simulink model "Blood_Pressure(Wrong)"  (R2024b)
settings: Solver=VariableStepAuto  StartTime=0.0  StopTime=10.0  RelTol=1e-3
values from neighbouring files (symbols this model uses):
  Ca = 87.5    [Blood_Pressure_Model.m]
  Co = 80    [Blood_Pressure_Model.m]
  MAP = 82.5    [Blood_Pressure_Model.m]
  VO2 = 37.5    [Blood_Pressure_Model.m]
undefined symbols (not defined in the file or in its folder): CVP
settings Model: Creator=Stephon Woodson  LastModifiedBy=Stephon Woodson

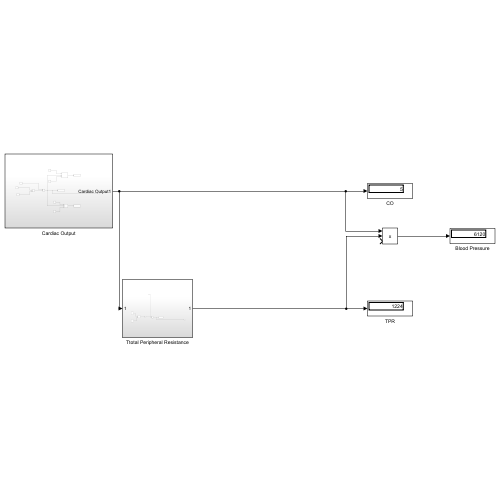
[thumbnail: Simulink's stored preview of the top-level diagram]
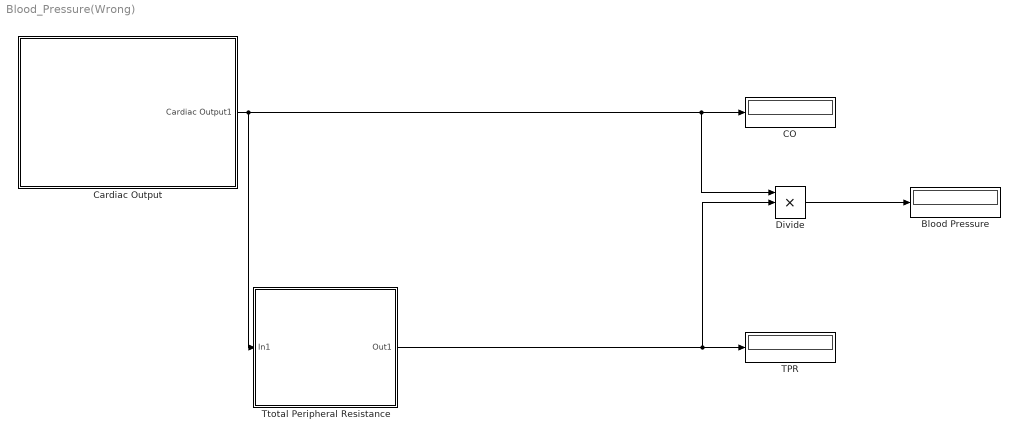
== system Blood_Pressure(Wrong) ==
  Blood Pressure : Display
  CO : Display
  Cardiac Output : Subsystem
  Divide : Product  Inputs=***
  TPR : Display
  Ttotal Peripheral Resistance : Subsystem
  wires:
  Cardiac Output/1(Cardiac Output1) -> Ttotal Peripheral Resistance/1(In1), Divide/1, CO/1
  Ttotal Peripheral Resistance/1(Out1) -> Divide/2, TPR/1
  Divide/1 -> Blood Pressure/1

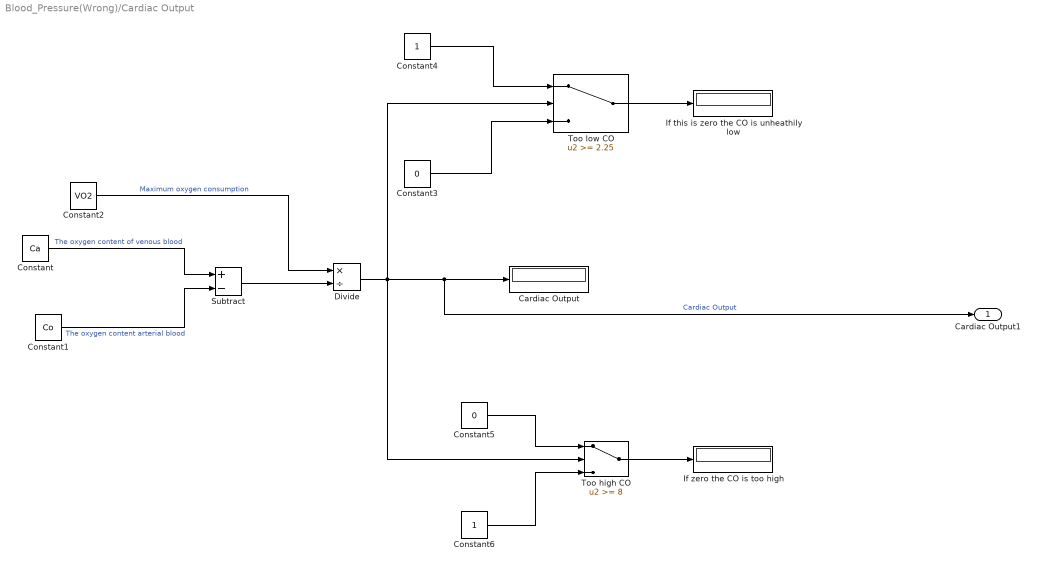
== system Blood_Pressure(Wrong)/Cardiac Output ==
  Cardiac Output : Display
  Constant : Constant  Value=Ca
  Constant1 : Constant  Value=Co
  Constant2 : Constant  Value=VO2
  Constant3 : Constant  Value=0
  Constant4 : Constant
  Constant5 : Constant  Value=0
  Constant6 : Constant
  Divide : Product  Inputs=*/
  If this is zero the CO is unheathily low : Display
  If zero the CO is too high : Display
  Subtract : Sum  Inputs=+-
  Too high CO : Switch  Threshold=8  SaturateOnIntegerOverflow=off  InputSameDT=off
  Too low CO : Switch  Threshold=2.25  SaturateOnIntegerOverflow=off  InputSameDT=off
  Cardiac Output1 : Outport
  wires:
  Constant1/1 -> Subtract/2  "The oxygen content arterial blood"
  Constant5/1 -> Too high CO/1
  Divide/1 -> Too high CO/2, Too low CO/2, Cardiac Output1/1, Cardiac Output/1  "Cardiac Output"
  Subtract/1 -> Divide/2
  Constant3/1 -> Too low CO/3
  Too high CO/1 -> If zero the CO is too high/1
  Constant/1 -> Subtract/1  "The oxygen content of venous blood"
  Constant2/1 -> Divide/1  "Maximum oxygen consumption"
  Constant6/1 -> Too high CO/3
  Too low CO/1 -> If this is zero the CO is unheathily low/1
  Constant4/1 -> Too low CO/1

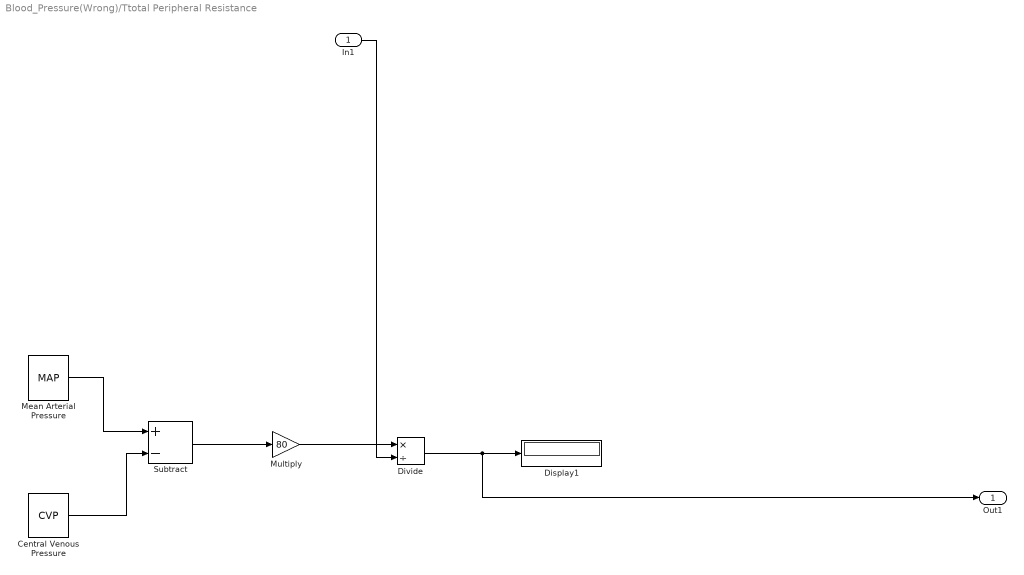
== system Blood_Pressure(Wrong)/Ttotal Peripheral Resistance ==
  In1 : Inport
  Central Venous Pressure : Constant  Value=CVP
  Display1 : Display
  Divide : Product  Inputs=*/
  Mean Arterial Pressure : Constant  Value=MAP
  Multiply : Gain  Gain=80
  Subtract : Sum  Inputs=+-
  Out1 : Outport
  wires:
  In1/1 -> Divide/2
  Mean Arterial Pressure/1 -> Subtract/1
  Subtract/1 -> Multiply/1
  Divide/1 -> Out1/1, Display1/1
  Central Venous Pressure/1 -> Subtract/2
  Multiply/1 -> Divide/1
